simulink model "homework6model"  (R2018a)
settings: Solver=ode5  StartTime=0.0  StopTime=200  RelTol=1e-3
settings Model: Creator=milos  LastModifiedBy=milos

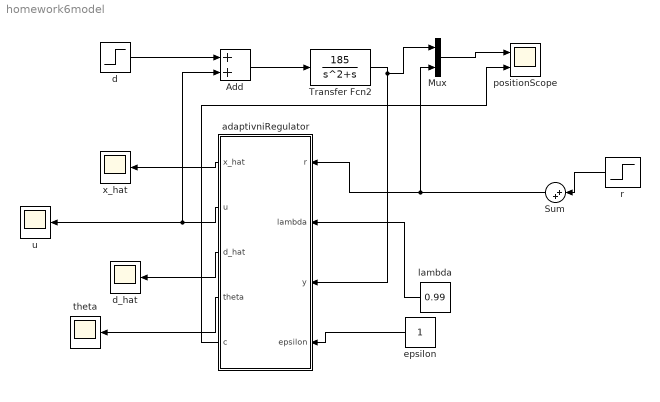
== system homework6model ==
  Add : Sum
  Mux : Mux  Inputs=2
  Sum : Sum  Inputs=|++
  Transfer Fcn2 : TransferFcn  Numerator=[185]  Denominator=[1 1 0]
  adaptivniRegulator : Subsystem
  d : Step  Time=20  After=0.5  SampleTime=0
  d_hat : Scope
  epsilon : Constant
  lambda : Constant  Value=0.99
  positionScope : Scope  NumInputPorts=2
  r : Step  Time=0  After=100  SampleTime=0
  theta : Scope
  u : Scope
  x_hat : Scope
  wires:
  Transfer Fcn2/1 -> Mux/1, adaptivniRegulator/3(y)
  Add/1 -> Transfer Fcn2/1
  d/1 -> Add/1
  r/1 -> Sum/1
  lambda/1 -> adaptivniRegulator/2(lambda)
  epsilon/1 -> adaptivniRegulator/4(epsilon)
  adaptivniRegulator/1(x_hat) -> x_hat/1
  adaptivniRegulator/2(u) -> Add/2, u/1
  adaptivniRegulator/3(d_hat) -> d_hat/1
  adaptivniRegulator/4(theta) -> theta/1
  Sum/1 -> Mux/2, adaptivniRegulator/1(r)
  Mux/1 -> positionScope/1
  adaptivniRegulator/5(c) -> positionScope/2

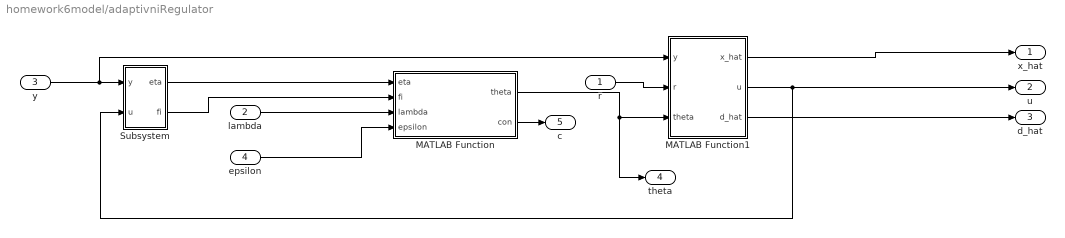
== system homework6model/adaptivniRegulator ==
  r : Inport
  lambda : Inport  Port=2
  y : Inport  Port=3
  epsilon : Inport  Port=4
  MATLAB Function : MATLAB Function  TreatAsAtomicUnit=on
  MATLAB Function1 : MATLAB Function  TreatAsAtomicUnit=on
  Subsystem : Subsystem
  x_hat : Outport
  u : Outport  Port=2
  d_hat : Outport  Port=3
  theta : Outport  Port=4
  c : Outport  Port=5
  wires:
  Subsystem/1(eta) -> MATLAB Function/1(eta)
  epsilon/1 -> MATLAB Function/4(epsilon)
  lambda/1 -> MATLAB Function/3(lambda)
  Subsystem/2(fi) -> MATLAB Function/2(fi)
  MATLAB Function/1(theta) -> theta/1, MATLAB Function1/3(theta)
  MATLAB Function1/3(d_hat) -> d_hat/1
  y/1 -> MATLAB Function1/1(y), Subsystem/1(y)
  MATLAB Function1/1(x_hat) -> x_hat/1
  r/1 -> MATLAB Function1/2(r)
  MATLAB Function1/2(u) -> Subsystem/2(u), u/1
  MATLAB Function/2(con) -> c/1

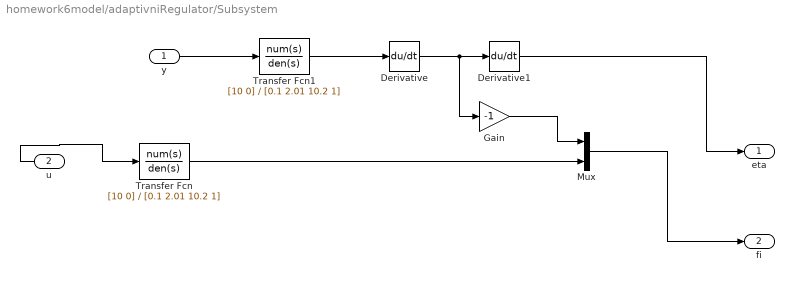
== system homework6model/adaptivniRegulator/Subsystem ==
  y : Inport
  u : Inport  Port=2
  Derivative : Derivative
  Derivative1 : Derivative
  Gain : Gain  Gain=-1
  Mux : Mux  Inputs=2
  Transfer Fcn : TransferFcn  Numerator=[10 0]  Denominator=[0.1 2.01 10.2 1]
  Transfer Fcn1 : TransferFcn  Numerator=[10 0]  Denominator=[0.1 2.01 10.2 1]
  eta : Outport
  fi : Outport  Port=2
  wires:
  Transfer Fcn1/1 -> Derivative/1
  u/1 -> Transfer Fcn/1
  Transfer Fcn/1 -> Mux/2
  Mux/1 -> fi/1
  Derivative1/1 -> eta/1
  Derivative/1 -> Gain/1, Derivative1/1
  Gain/1 -> Mux/1
  y/1 -> Transfer Fcn1/1

== matlab function homework6model/adaptivniRegulator/MATLAB Function1 ==
  settings: updateMethod=DISCRETE  sampleTime=0.01
  data: y input; x_hat output; r input; u output; d_hat output; T parameter; theta input
function [x_hat,u,d_hat] = regulator(y,r,T, theta)
persistent  x_hat_p;
persistent w_hat_p;
persistent i;
if isempty(x_hat_p) || isempty(w_hat_p)
    x_hat_p=[0;0];
    w_hat_p=0;
    i=0;
end

A=[0 1;0 ,-theta(1)];
B=[0;theta(2)];
C=[1 0];

Aw=0;
Cw=1;

Td=1;
a=1/Td;
Acls=poly([-a,-a]);
% calculate gains of regulator
k1=Acls(end)/B(2);
k2=(Acls(end-1)+A(2,2))/B(2);
k=[k1,k2];

%create model including disturbance 
Asd=[A , B*Cw; zeros(size(Aw,1),size(A,1)), Aw];
Bsd=[B;zeros(size(Aw,1),size(B,2))];
Csd=[C,zeros(1,size(Aw,1))];

% chose poles
pole=-4*ones(1,size(Asd,1));
Acl=poly(pole);
% calculate observer gains
%L=acker(Asd',Csd',pole)';
l3=Acl(end)/Asd(2,3);
l1=Acl(end-2)+Asd(2,2);
l2=Acl(end-1)+Asd(2,2)*l1;
Lw=l3;
L=[l1;l2];

swN=0; % 1-noise
swD=1; % 1- contant disturbance, 2-ramp , 3-periodic

kr=k(1);

d_hat=Cw*w_hat_p;
%if i*T<3
    %u=0.5;
%else
u=-k*x_hat_p+kr*r-d_hat;
if u>1
    u=1;
elseif u<-1
    u=-1;
end
%end
i=i+1;
x_hat=x_hat_p+T*(A*x_hat_p+B*(u+d_hat)+L*(y-C*x_hat_p));
w_hat_p=w_hat_p+T*(Aw*w_hat_p+Lw*(y-C*x_hat_p));
x_hat_p=x_hat;
if isnan(w_hat_p)
    s=1;
end
end

== matlab function homework6model/adaptivniRegulator/MATLAB Function ==
  settings: updateMethod=DISCRETE  sampleTime=10*T
  data: eta input; theta output; fi input; lambda input; epsilon input; con output
function [theta,con]  =recursive_least_squeres(eta,fi,lambda,epsilon)
persistent theta_p
persistent P_p
if isempty(theta_p)
    theta_p=0.1*ones(size(fi));
    P_p=1000*eye(size(fi,1));
end
con=fi'*P_p*fi > epsilon*(1-lambda);
if con
   P=1/lambda*(P_p-P_p*fi * fi'*P_p/ (lambda+fi'*P_p*fi));
   err=eta-fi'*theta_p;
   theta=theta_p+P*fi*(err);
   theta_p=theta;
   P_p=P;
else
    theta=theta_p;
end
